simulink model "Ctrl_For_HRV"  (R2024b)
settings: Solver=ode4  StartTime=0.0  StopTime=100  FixedStep=0.02  RelTol=1e-3
InitFcn:
  | Parameter;
undefined symbols (not defined in the file or in its folder): CCI_DUI_AngleRate_Controller, CCI_DUI_FlowAngle_Controller, fhan, h_alpha, h_beta, h_miu, h_p, h_q, h_r, PNG_2026_6_24, r_alpha, r_beta, r_miu, r_p, r_q, r_r, xishu, xishu_D_0, xishu_L_0, xishu_l_0, xishu_m_0, xishu_n_0, xishu_Y_0
libraries: simulink x12
settings Model: Creator=BinRen  LastModifiedBy=DuY
settings SolverCC: AlgebraicLoopSolver=TrustRegion
settings DataIOCC: ReturnWorkspaceOutputs=off  TimeSaveName=time
settings DebuggingCC: UnconnectedInputMsg=warning  UnconnectedOutputMsg=warning  UnconnectedLineMsg=warning
settings ModelReferenceCC: EnableRefExpFcnMdlSchedulingChecks=on
settings RTWCC: GPUComputeCapability=3.5  DLArmComputeVersion=19.05

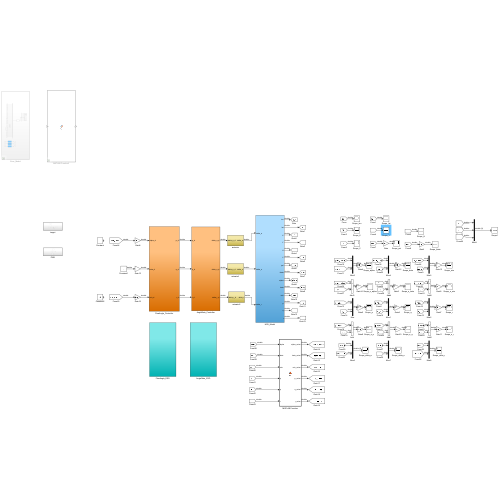
[thumbnail: Simulink's stored preview of the top-level diagram]
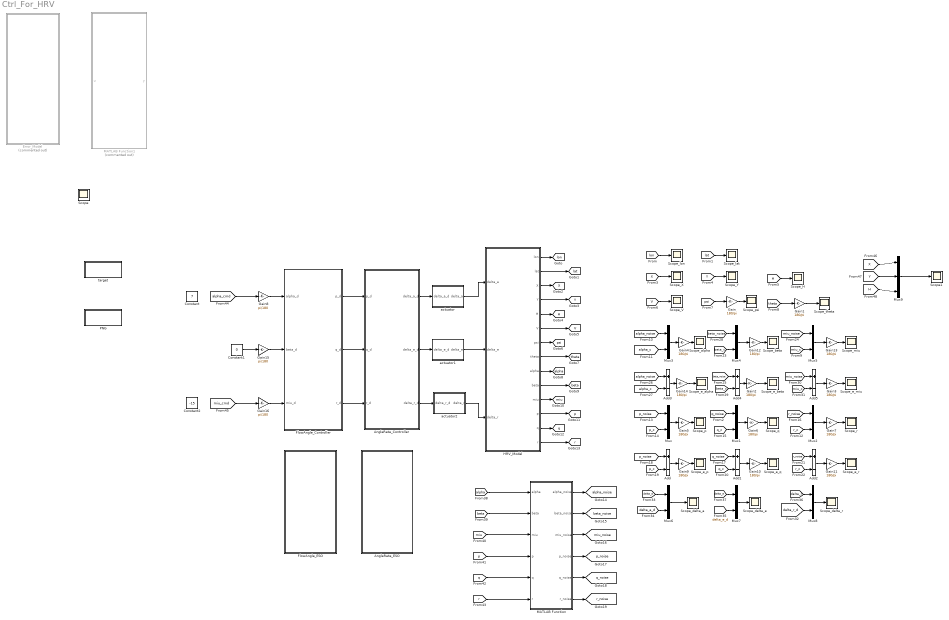
== system Ctrl_For_HRV ==
  Add{,1..5} (6 alike) : Sum  Inputs=+-
  AngleRate_Controller : Subsystem
  AngleRate_ESO : Subsystem
  Constant : Constant  Value=7  SampleTime=-1
  Constant1 : Constant  Value=0  SampleTime=-1
  Constant2 : Constant  Value=-15  SampleTime=-1
  Error_Model : Subsystem  Commented=on
  FlowAngle_Controller : Subsystem
  FlowAngle_ESO : Subsystem
  Gain{,1..7,9..14} (14 alike) : Gain  Gain=180/pi
  Gain15 : Gain  Gain=pi/180
  Gain16 : Gain  Gain=pi/180
  Gain8 : Gain  Gain=pi/180
  HRV_Model : Subsystem
  MATLAB Function : MATLAB Function  TreatAsAtomicUnit=on
  MATLAB Function1 : MATLAB Function  Commented=on  TreatAsAtomicUnit=on
  Mux{,1..8} (9 alike) : Mux  Inputs=2
  Mux9 : Mux  Inputs=3
  PNG : Subsystem
  Scope1 : Scope
  Scope_H : Scope
  Scope_V : Scope
  Scope_X : Scope
  Scope_Y : Scope
  Scope_alpha : Scope
  Scope_beta : Scope
  Scope_delta_a : Scope
  Scope_delta_e : Scope
  Scope_delta_r : Scope
  Scope_e_alpha : Scope
  Scope_e_beta : Scope
  Scope_e_miu : Scope
  Scope_e_p : Scope
  Scope_e_q : Scope
  Scope_e_r : Scope
  Scope_lat : Scope
  Scope_lon : Scope
  Scope_miu : Scope
  Scope_p : Scope
  Scope_psi : Scope
  Scope_q : Scope
  Scope_r : Scope
  Scope_theta : Scope
  actuator : Subsystem
  actuator1 : Subsystem
  actuator2 : Subsystem
  target : Subsystem
  Scope : Scope
  tag scope: H=global, V=global, X=global, Y=global, alpha=global, alpha_noise=global, beta=global, beta_noise=global, lat=global, lon=global, miu=global, miu_noise=global, p=global, p_noise=global, psi=global, q=global, q_noise=global, r=global, r_noise=global, theta=global
  wires:
  HRV_Model/1(lon) -> [lon]
  HRV_Model/2(lat) -> [lat]
  HRV_Model/4(Y) -> [Y]
  HRV_Model/3(X) -> [X]
  HRV_Model/7(psi) -> [psi]
  HRV_Model/8(theta) -> [theta]
  HRV_Model/6(V) -> [V]
  HRV_Model/5(H) -> [H]
  HRV_Model/13(q) -> [q]
  HRV_Model/14(r) -> [r]
  HRV_Model/11(miu) -> [miu]
  HRV_Model/12(p) -> [p]
  HRV_Model/10(beta) -> [beta]
  HRV_Model/9(alpha) -> [alpha]
  [lon] -> Scope_lon/1
  [lat] -> Scope_lat/1
  [H] -> Scope_H/1
  [Y] -> Scope_Y/1
  [X] -> Scope_X/1
  [V] -> Scope_V/1
  [psi] -> Gain/1
  Gain/1 -> Scope_psi/1
  Gain1/1 -> Scope_theta/1
  [theta] -> Gain1/1
  Gain5/1 -> Scope_p/1
  Gain6/1 -> Scope_q/1
  Gain7/1 -> Scope_r/1
  actuator/1(delta_a) -> HRV_Model/1(delta_a)
  actuator1/1(delta_e) -> HRV_Model/2(delta_e)
  actuator2/1(delta_r) -> HRV_Model/3(delta_r)
  AngleRate_Controller/2(delta_e_d) -> actuator1/1(delta_e_d)
  [p_noise] -> Mux/1
  Mux/1 -> Gain5/1
  [p_c] -> Mux/2
  [q_c] -> Mux1/2
  [q_noise] -> Mux1/1
  Mux1/1 -> Gain6/1
  Mux2/1 -> Gain7/1
  [r_noise] -> Mux2/1
  [r_c] -> Mux2/2
  Gain11/1 -> Scope_e_r/1
  Gain10/1 -> Scope_e_q/1
  Gain9/1 -> Scope_e_p/1
  [p_c] -> Add/2
  [p_noise] -> Add/1
  Add/1 -> Gain9/1
  Add1/1 -> Gain10/1
  [q_noise] -> Add1/1
  [q_c] -> Add1/2
  [r_c] -> Add2/2
  [r_noise] -> Add2/1
  Add2/1 -> Gain11/1
  Add5/1 -> Gain3/1
  [miu_noise] -> Add5/1
  [miu_c] -> Add5/2
  [beta_c] -> Add4/2
  [beta_noise] -> Add4/1
  Add4/1 -> Gain2/1
  Add3/1 -> Gain14/1
  [alpha_noise] -> Add3/1
  [alpha_c] -> Add3/2
  Gain14/1 -> Scope_e_alpha/1
  Gain2/1 -> Scope_e_beta/1
  Gain3/1 -> Scope_e_miu/1
  [miu_c] -> Mux5/2
  [miu_noise] -> Mux5/1
  Mux5/1 -> Gain13/1
  Mux4/1 -> Gain12/1
  [beta_noise] -> Mux4/1
  [beta_c] -> Mux4/2
  [alpha_c] -> Mux3/2
  Mux3/1 -> Gain4/1
  [alpha_noise] -> Mux3/1
  Gain13/1 -> Scope_miu/1
  Gain12/1 -> Scope_beta/1
  Gain4/1 -> Scope_alpha/1
  Gain8/1 -> FlowAngle_Controller/1(alpha_d)
  [delta_r_d] -> Mux8/2
  [delta_r] -> Mux8/1
  [delta_e] -> Mux7/1
  [delta_e_d] -> Mux7/2
  [delta_a_d] -> Mux6/2
  [delta_a] -> Mux6/1
  Mux8/1 -> Scope_delta_r/1
  Mux7/1 -> Scope_delta_e/1
  Mux6/1 -> Scope_delta_a/1
  FlowAngle_Controller/1(p_d) -> AngleRate_Controller/1(p_d)
  FlowAngle_Controller/2(q_d) -> AngleRate_Controller/2(q_d)
  FlowAngle_Controller/3(r_d) -> AngleRate_Controller/3(r_d)
  Constant1/1 -> Gain15/1
  Gain15/1 -> FlowAngle_Controller/2(beta_d)
  Gain16/1 -> FlowAngle_Controller/3(miu_d)
  AngleRate_Controller/3(delta_r_d) -> actuator2/1(delta_r_d)
  AngleRate_Controller/1(delta_a_d) -> actuator/1(delta_a_d)
  MATLAB Function/1(alpha_noise) -> [alpha_noise]
  [alpha] -> MATLAB Function/1(alpha)
  [beta] -> MATLAB Function/2(beta)
  [miu] -> MATLAB Function/3(miu)
  [p] -> MATLAB Function/4(p)
  [q] -> MATLAB Function/5(q)
  [r] -> MATLAB Function/6(r)
  MATLAB Function/2(beta_noise) -> [beta_noise]
  MATLAB Function/3(miu_noise) -> [miu_noise]
  MATLAB Function/4(p_noise) -> [p_noise]
  MATLAB Function/5(q_noise) -> [q_noise]
  MATLAB Function/6(r_noise) -> [r_noise]
  [miu_cmd] -> Gain16/1
  [alpha_cmd] -> Gain8/1
  [X] -> Mux9/1
  [Y] -> Mux9/2
  [H] -> Mux9/3
  Mux9/1 -> Scope1/1

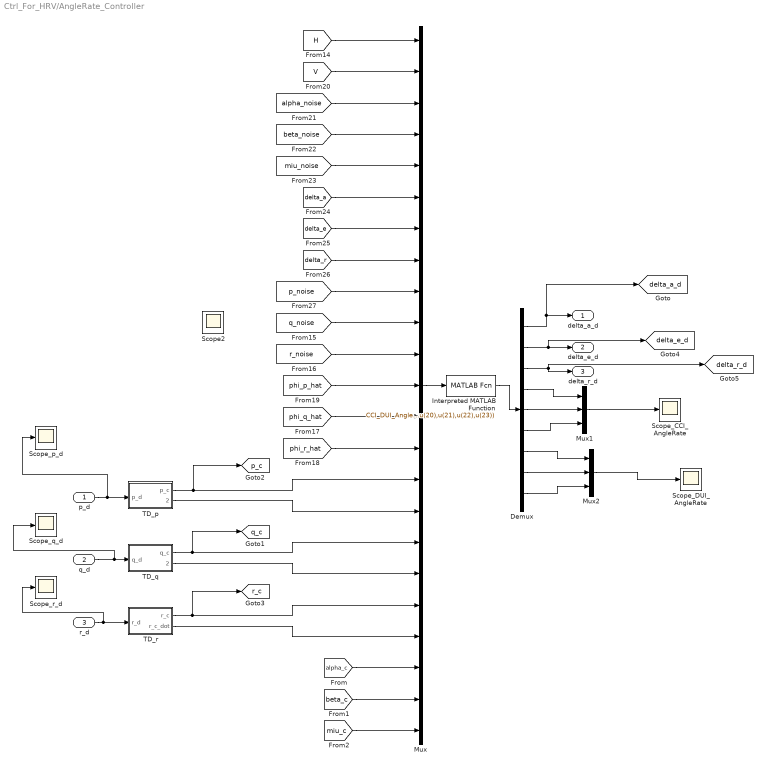
== system Ctrl_For_HRV/AngleRate_Controller ==
  p_d : Inport
  q_d : Inport  Port=2
  r_d : Inport  Port=3
  Demux : Demux  Outputs=9
  Interpreted MATLAB Function : MATLABFcn  MATLABFcn=CCI_DUI_AngleRate_Controller(u(1),u(2),u(3),u(4),u(5),u(6),u(7),u(8),u(9),u(10),u(11),u(12),u(13),u(14),u(15),u(16),u(17),u(18),u(19),u(20),u(21),u(22),u(23))  OutputDimensions=9
  Mux : Mux  Inputs=23
  Mux1 : Mux  Inputs=3
  Mux2 : Mux  Inputs=3
  Scope2 : Scope
  Scope_CCI_AngleRate : Scope
  Scope_DUI_AngleRate : Scope
  Scope_p_d : Scope
  Scope_q_d : Scope
  Scope_r_d : Scope
  TD_p : Subsystem
  TD_q : Subsystem
  TD_r : Subsystem
  delta_a_d : Outport
  delta_e_d : Outport  Port=2
  delta_r_d : Outport  Port=3
  tag scope: delta_a_d=global, delta_e_d=global, delta_r_d=global, p_c=global, q_c=global, r_c=global
  wires:
  [miu_noise] -> Mux/5
  [beta_noise] -> Mux/4
  TD_r/1(r_c) -> [r_c], Mux/19
  TD_p/2(p_c_dot) -> Mux/16
  TD_q/2(q_c_dot) -> Mux/18
  [q_noise] -> Mux/10
  TD_q/1(q_c) -> [q_c], Mux/17
  TD_r/2(r_c_dot) -> Mux/20
  [r_noise] -> Mux/11
  [H] -> Mux/1
  [p_noise] -> Mux/9
  [V] -> Mux/2
  [alpha_noise] -> Mux/3
  Mux/1 -> Interpreted MATLAB Function/1
  Interpreted MATLAB Function/1 -> Demux/1
  [delta_a] -> Mux/6
  [delta_r] -> Mux/8
  [delta_e] -> Mux/7
  TD_p/1(p_c) -> [p_c], Mux/15
  Demux/3 -> delta_r_d/1, [delta_r_d]
  r_d/1 -> Scope_r_d/1, TD_r/1(r_d)
  Demux/2 -> [delta_e_d], delta_e_d/1
  Demux/1 -> [delta_a_d], delta_a_d/1
  q_d/1 -> Scope_q_d/1, TD_q/1(q_d)
  p_d/1 -> Scope_p_d/1, TD_p/1(p_d)
  [phi_p_hat] -> Mux/12
  [phi_q_hat] -> Mux/13
  [phi_r_hat] -> Mux/14
  [alpha_c] -> Mux/21
  [beta_c] -> Mux/22
  [miu_c] -> Mux/23
  Demux/4 -> Mux1/1
  Demux/5 -> Mux1/2
  Demux/6 -> Mux1/3
  Mux1/1 -> Scope_CCI_AngleRate/1
  Demux/7 -> Mux2/1
  Demux/8 -> Mux2/2
  Demux/9 -> Mux2/3
  Mux2/1 -> Scope_DUI_AngleRate/1

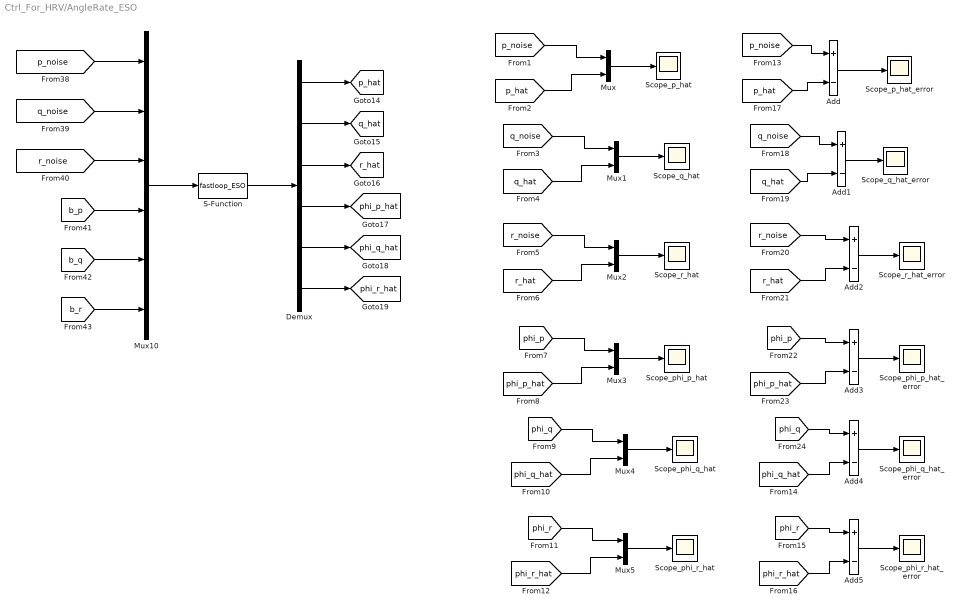
== system Ctrl_For_HRV/AngleRate_ESO ==
  Add{,1..5} (6 alike) : Sum  Inputs=+-
  Demux : Demux  Outputs=6
  Mux{,1..5} (6 alike) : Mux  Inputs=2
  Mux10 : Mux  Inputs=6
  S-Function : S-Function  FunctionName=fastloop_ESO  SFunctionDeploymentMode=off  EnableBusSupport=off
  Scope_p_hat : Scope
  Scope_p_hat_error : Scope
  Scope_phi_p_hat : Scope
  Scope_phi_p_hat_error : Scope
  Scope_phi_q_hat : Scope
  Scope_phi_q_hat_error : Scope
  Scope_phi_r_hat : Scope
  Scope_phi_r_hat_error : Scope
  Scope_q_hat : Scope
  Scope_q_hat_error : Scope
  Scope_r_hat : Scope
  Scope_r_hat_error : Scope
  tag scope: p_hat=global, phi_p_hat=global, phi_q_hat=global, phi_r_hat=global, q_hat=global, r_hat=global
  wires:
  [b_q] -> Mux10/5
  [r_noise] -> Mux10/3
  [q_noise] -> Mux10/2
  Demux/2 -> [q_hat]
  [b_p] -> Mux10/4
  S-Function/1 -> Demux/1
  Demux/5 -> [phi_q_hat]
  Demux/1 -> [p_hat]
  Demux/3 -> [r_hat]
  Demux/4 -> [phi_p_hat]
  Mux10/1 -> S-Function/1
  Demux/6 -> [phi_r_hat]
  [p_noise] -> Mux10/1
  [b_r] -> Mux10/6
  Mux/1 -> Scope_p_hat/1
  [p_noise] -> Mux/1
  [p_hat] -> Mux/2
  [q_noise] -> Mux1/1
  [q_hat] -> Mux1/2
  Mux1/1 -> Scope_q_hat/1
  [r_noise] -> Mux2/1
  [r_hat] -> Mux2/2
  Mux2/1 -> Scope_r_hat/1
  Mux5/1 -> Scope_phi_r_hat/1
  [phi_r_hat] -> Mux5/2
  [phi_r] -> Mux5/1
  Mux4/1 -> Scope_phi_q_hat/1
  [phi_q_hat] -> Mux4/2
  [phi_q] -> Mux4/1
  [phi_p_hat] -> Mux3/2
  [phi_p] -> Mux3/1
  Mux3/1 -> Scope_phi_p_hat/1
  [p_noise] -> Add/1
  [p_hat] -> Add/2
  Add/1 -> Scope_p_hat_error/1
  [q_noise] -> Add1/1
  [q_hat] -> Add1/2
  Add1/1 -> Scope_q_hat_error/1
  [r_noise] -> Add2/1
  [r_hat] -> Add2/2
  Add2/1 -> Scope_r_hat_error/1
  [phi_p] -> Add3/1
  [phi_p_hat] -> Add3/2
  Add3/1 -> Scope_phi_p_hat_error/1
  [phi_q] -> Add4/1
  [phi_q_hat] -> Add4/2
  Add4/1 -> Scope_phi_q_hat_error/1
  [phi_r] -> Add5/1
  [phi_r_hat] -> Add5/2
  Add5/1 -> Scope_phi_r_hat_error/1

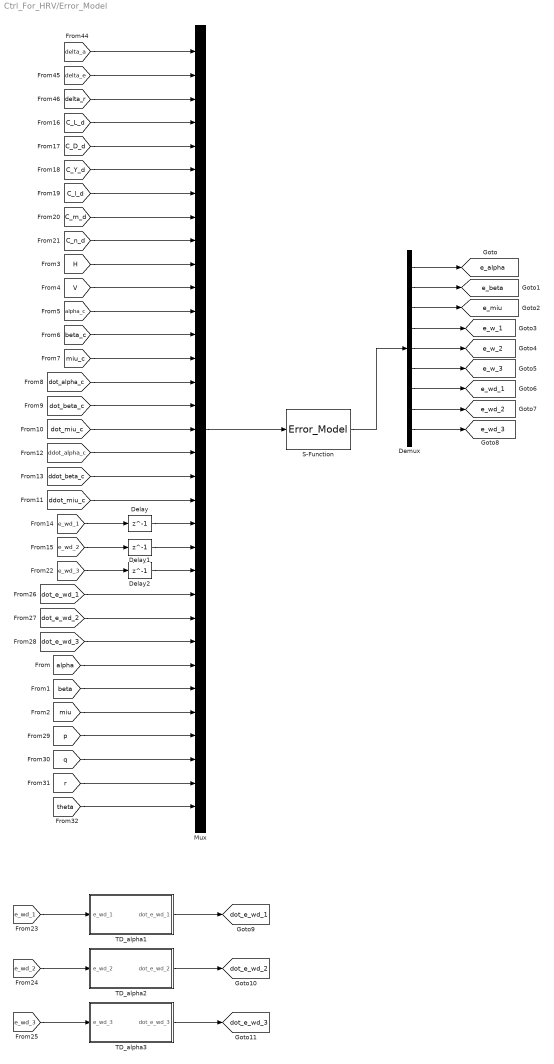
== system Ctrl_For_HRV/Error_Model ==
  Delay : Delay  DelayLength=1
  Delay1 : Delay  DelayLength=1
  Delay2 : Delay  DelayLength=1
  Demux : Demux  Outputs=9
  Mux : Mux  Inputs=33
  S-Function : S-Function  FunctionName=Error_Model  SFunctionDeploymentMode=off  EnableBusSupport=off
  TD_alpha1 : Subsystem
  TD_alpha2 : Subsystem
  TD_alpha3 : Subsystem
  tag scope: dot_e_wd_1=global, dot_e_wd_2=global, dot_e_wd_3=global, e_alpha=global, e_beta=global, e_miu=global, e_w_1=global, e_w_2=global, e_w_3=global, e_wd_1=global, e_wd_2=global, e_wd_3=global
  wires:
  Mux/1 -> S-Function/1
  [C_l_d] -> Mux/7
  [C_D_d] -> Mux/5
  [C_L_d] -> Mux/4
  [C_Y_d] -> Mux/6
  [C_n_d] -> Mux/9
  [C_m_d] -> Mux/8
  [H] -> Mux/10
  [V] -> Mux/11
  [alpha_c] -> Mux/12
  [beta_c] -> Mux/13
  [miu_c] -> Mux/14
  [dot_miu_c] -> Mux/17
  [dot_beta_c] -> Mux/16
  [dot_alpha_c] -> Mux/15
  [ddot_alpha_c] -> Mux/18
  [ddot_beta_c] -> Mux/19
  [ddot_miu_c] -> Mux/20
  S-Function/1 -> Demux/1
  Demux/1 -> [e_alpha]
  Demux/2 -> [e_beta]
  Demux/3 -> [e_miu]
  Demux/4 -> [e_w_1]
  Demux/5 -> [e_w_2]
  Demux/6 -> [e_w_3]
  Demux/9 -> [e_wd_3]
  Demux/8 -> [e_wd_2]
  Demux/7 -> [e_wd_1]
  [e_wd_1] -> Delay/1
  Delay/1 -> Mux/21
  Delay1/1 -> Mux/22
  [e_wd_2] -> Delay1/1
  [e_wd_3] -> Delay2/1
  Delay2/1 -> Mux/23
  [e_wd_1] -> TD_alpha1/1(e_wd_1)
  TD_alpha1/1(dot_e_wd_1) -> [dot_e_wd_1]
  TD_alpha2/1(dot_e_wd_2) -> [dot_e_wd_2]
  [e_wd_2] -> TD_alpha2/1(e_wd_2)
  [e_wd_3] -> TD_alpha3/1(e_wd_3)
  TD_alpha3/1(dot_e_wd_3) -> [dot_e_wd_3]
  [dot_e_wd_1] -> Mux/24
  [dot_e_wd_2] -> Mux/25
  [dot_e_wd_3] -> Mux/26
  [delta_a] -> Mux/1
  [delta_e] -> Mux/2
  [delta_r] -> Mux/3
  [alpha] -> Mux/27
  [beta] -> Mux/28
  [miu] -> Mux/29
  [p] -> Mux/30
  [q] -> Mux/31
  [r] -> Mux/32
  [theta] -> Mux/33

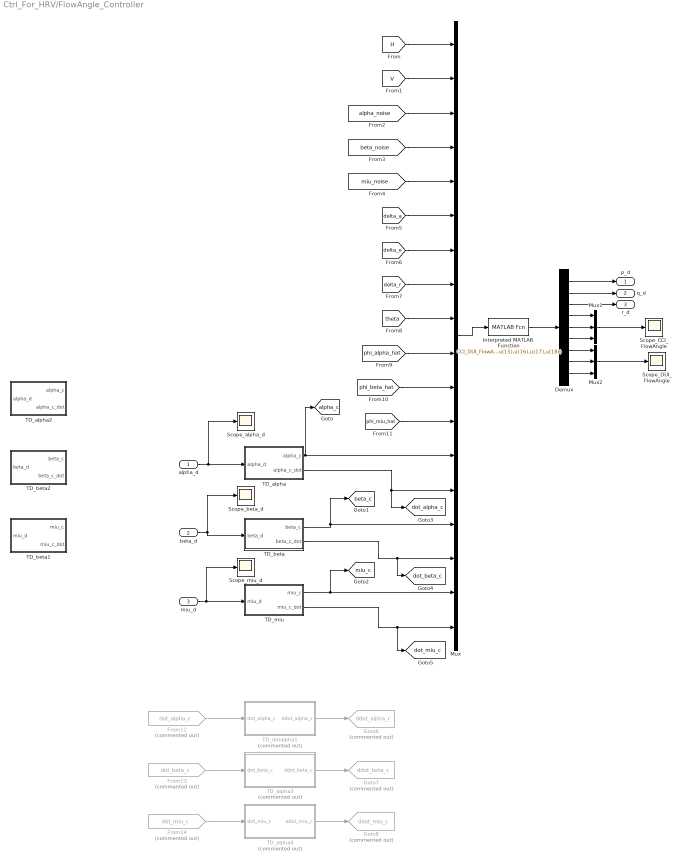
== system Ctrl_For_HRV/FlowAngle_Controller ==
  alpha_d : Inport
  beta_d : Inport  Port=2
  miu_d : Inport  Port=3
  Demux : Demux  Outputs=9
  From12 : From  Commented=on  GotoTag=dot_alpha_c  TagVisibility=global
  From13 : From  Commented=on  GotoTag=dot_beta_c  TagVisibility=global
  From14 : From  Commented=on  GotoTag=dot_miu_c  TagVisibility=global
  Goto6 : Goto  Commented=on  GotoTag=ddot_alpha_c  TagVisibility=global
  Goto7 : Goto  Commented=on  GotoTag=ddot_beta_c  TagVisibility=global
  Goto8 : Goto  Commented=on  GotoTag=ddot_miu_c  TagVisibility=global
  Interpreted MATLAB Function : MATLABFcn  MATLABFcn=CCI_DUI_FlowAngle_Controller(u(1),u(2),u(3),u(4),u(5),u(6),u(7),u(8),u(9),u(10),u(11),u(12),u(13),u(14),u(15),u(16),u(17),u(18))  OutputDimensions=9
  Mux : Mux  Inputs=18
  Mux1 : Mux  Inputs=3
  Mux2 : Mux  Inputs=3
  Scope_CCI_FlowAngle : Scope
  Scope_DUI_FlowAngle : Scope
  Scope_alpha_d : Scope
  Scope_beta_d : Scope
  Scope_miu_d : Scope
  TD_alpha : Subsystem
  TD_alpha2 : Subsystem
  TD_alpha3 : Subsystem  Commented=on
  TD_alpha4 : Subsystem  Commented=on
  TD_beta : Subsystem
  TD_beta1 : Subsystem
  TD_beta2 : Subsystem
  TD_dotalpha1 : Subsystem  Commented=on
  TD_miu : Subsystem
  p_d : Outport
  q_d : Outport  Port=2
  r_d : Outport  Port=3
  tag scope: alpha_c=global, beta_c=global, dot_alpha_c=global, dot_beta_c=global, dot_miu_c=global, miu_c=global
  wires:
  [H] -> Mux/1
  [V] -> Mux/2
  [alpha_noise] -> Mux/3
  [beta_noise] -> Mux/4
  [miu_noise] -> Mux/5
  [delta_r] -> Mux/8
  [delta_e] -> Mux/7
  [delta_a] -> Mux/6
  [theta] -> Mux/9
  Mux/1 -> Interpreted MATLAB Function/1
  Interpreted MATLAB Function/1 -> Demux/1
  Demux/1 -> p_d/1
  Demux/2 -> q_d/1
  Demux/3 -> r_d/1
  alpha_d/1 -> Scope_alpha_d/1, TD_alpha/1(alpha_d)
  TD_alpha/2(alpha_c_dot) -> Mux/14, [dot_alpha_c]
  beta_d/1 -> Scope_beta_d/1, TD_beta/1(beta_d)
  TD_beta/1(beta_c) -> [beta_c], Mux/15
  TD_beta/2(beta_c_dot) -> [dot_beta_c], Mux/16
  miu_d/1 -> Scope_miu_d/1, TD_miu/1(miu_d)
  TD_miu/1(miu_c) -> [miu_c], Mux/17
  TD_miu/2(miu_c_dot) -> [dot_miu_c], Mux/18
  [phi_alpha_hat] -> Mux/10
  [phi_beta_hat] -> Mux/11
  [phi_miu_hat] -> Mux/12
  From12/1 -> TD_dotalpha1/1(dot_alpha_c)
  TD_dotalpha1/1(ddot_alpha_c) -> Goto6/1
  From13/1 -> TD_alpha3/1(dot_beta_c)
  TD_alpha3/1(ddot_beta_c) -> Goto7/1
  From14/1 -> TD_alpha4/1(dot_miu_c)
  TD_alpha4/1(ddot_miu_c) -> Goto8/1
  TD_alpha/1(alpha_c) -> [alpha_c], Mux/13
  Demux/4 -> Mux1/1
  Demux/5 -> Mux1/2
  Demux/6 -> Mux1/3
  Mux1/1 -> Scope_CCI_FlowAngle/1
  Mux2/1 -> Scope_DUI_FlowAngle/1
  Demux/8 -> Mux2/2
  Demux/9 -> Mux2/3
  Demux/7 -> Mux2/1

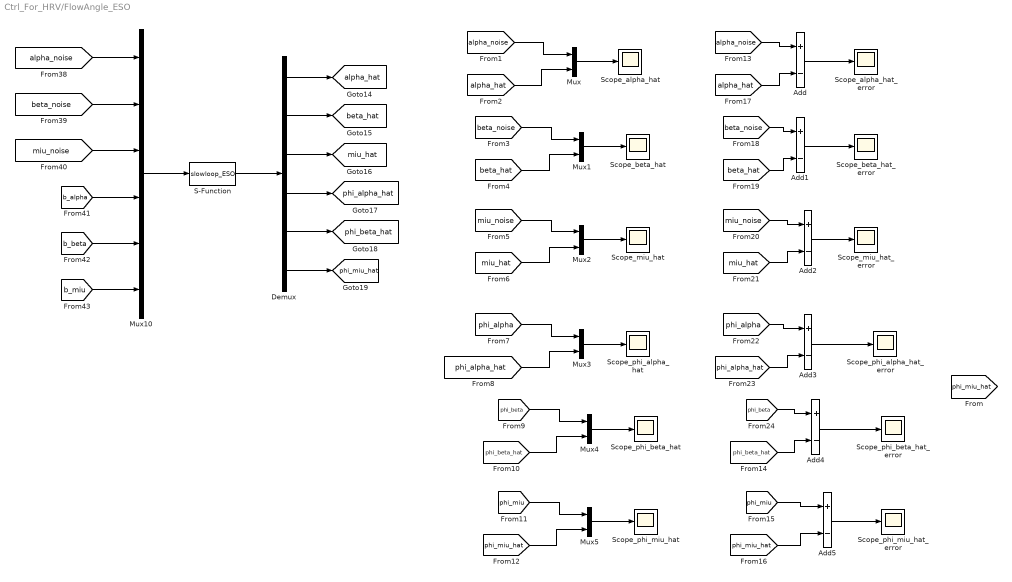
== system Ctrl_For_HRV/FlowAngle_ESO ==
  Add{,1..5} (6 alike) : Sum  Inputs=+-
  Demux : Demux  Outputs=6
  Mux{,1..5} (6 alike) : Mux  Inputs=2
  Mux10 : Mux  Inputs=6
  S-Function : S-Function  FunctionName=slowloop_ESO  SFunctionDeploymentMode=off  EnableBusSupport=off
  Scope_alpha_hat : Scope
  Scope_alpha_hat_error : Scope
  Scope_beta_hat : Scope
  Scope_beta_hat_error : Scope
  Scope_miu_hat : Scope
  Scope_miu_hat_error : Scope
  Scope_phi_alpha_hat : Scope
  Scope_phi_alpha_hat_error : Scope
  Scope_phi_beta_hat : Scope
  Scope_phi_beta_hat_error : Scope
  Scope_phi_miu_hat : Scope
  Scope_phi_miu_hat_error : Scope
  tag scope: alpha_hat=global, beta_hat=global, miu_hat=global, phi_alpha_hat=global, phi_beta_hat=global, phi_miu_hat=global
  wires:
  [b_beta] -> Mux10/5
  [miu_noise] -> Mux10/3
  [beta_noise] -> Mux10/2
  Demux/2 -> [beta_hat]
  [b_alpha] -> Mux10/4
  S-Function/1 -> Demux/1
  Demux/5 -> [phi_beta_hat]
  Demux/1 -> [alpha_hat]
  Demux/3 -> [miu_hat]
  Demux/4 -> [phi_alpha_hat]
  Mux10/1 -> S-Function/1
  Demux/6 -> [phi_miu_hat]
  [alpha_noise] -> Mux10/1
  [b_miu] -> Mux10/6
  Mux/1 -> Scope_alpha_hat/1
  [alpha_noise] -> Mux/1
  [alpha_hat] -> Mux/2
  [beta_noise] -> Mux1/1
  [beta_hat] -> Mux1/2
  Mux1/1 -> Scope_beta_hat/1
  [miu_noise] -> Mux2/1
  [miu_hat] -> Mux2/2
  Mux2/1 -> Scope_miu_hat/1
  Mux5/1 -> Scope_phi_miu_hat/1
  [phi_miu_hat] -> Mux5/2
  [phi_miu] -> Mux5/1
  Mux4/1 -> Scope_phi_beta_hat/1
  [phi_beta_hat] -> Mux4/2
  [phi_beta] -> Mux4/1
  [phi_alpha_hat] -> Mux3/2
  [phi_alpha] -> Mux3/1
  Mux3/1 -> Scope_phi_alpha_hat/1
  [alpha_noise] -> Add/1
  [alpha_hat] -> Add/2
  Add/1 -> Scope_alpha_hat_error/1
  [beta_noise] -> Add1/1
  [beta_hat] -> Add1/2
  Add1/1 -> Scope_beta_hat_error/1
  [miu_noise] -> Add2/1
  [miu_hat] -> Add2/2
  Add2/1 -> Scope_miu_hat_error/1
  [phi_alpha] -> Add3/1
  [phi_alpha_hat] -> Add3/2
  Add3/1 -> Scope_phi_alpha_hat_error/1
  [phi_beta] -> Add4/1
  [phi_beta_hat] -> Add4/2
  Add4/1 -> Scope_phi_beta_hat_error/1
  Add5/1 -> Scope_phi_miu_hat_error/1
  [phi_miu] -> Add5/1
  [phi_miu_hat] -> Add5/2

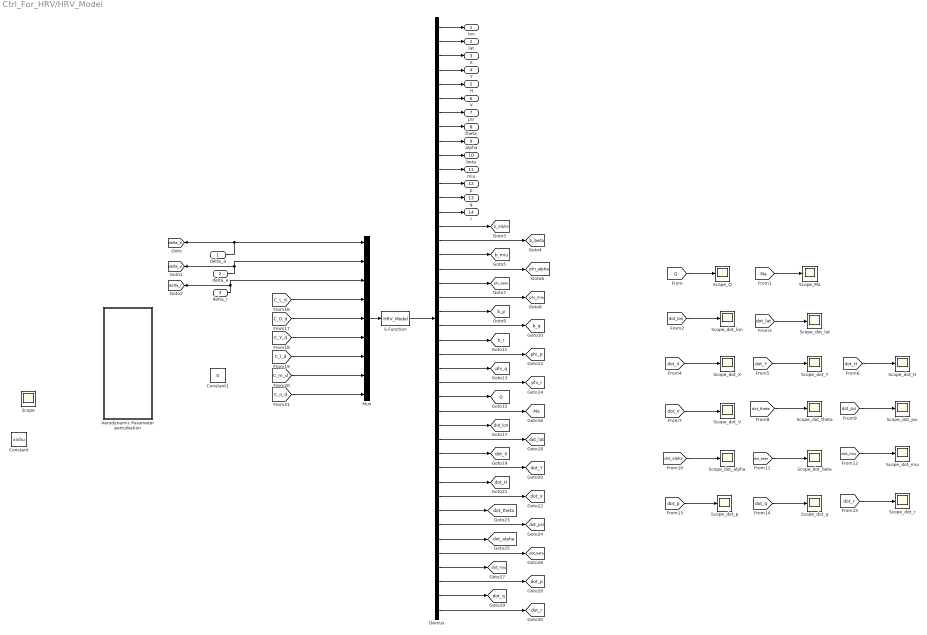
== system Ctrl_For_HRV/HRV_Model ==
  delta_a : Inport
  delta_e : Inport  Port=2
  delta_r : Inport  Port=3
  Aerodynamic Parameter perturbation : Subsystem
  Constant : Constant  Value=xishu  SampleTime=-1
  Constant1 : Constant  Value=0
  Demux : Demux  Outputs=14 + 12 + 2 + 14
  Mux : Mux  Inputs=9
  S-Function : S-Function  FunctionName=HRV_Model  SFunctionDeploymentMode=off  EnableBusSupport=off
  Scope : Scope
  Scope_Ma : Scope
  Scope_Q : Scope
  Scope_dot_H : Scope
  Scope_dot_V : Scope
  Scope_dot_X : Scope
  Scope_dot_Y : Scope
  Scope_dot_alpha : Scope
  Scope_dot_beta : Scope
  Scope_dot_lat : Scope
  Scope_dot_lon : Scope
  Scope_dot_miu : Scope
  Scope_dot_p : Scope
  Scope_dot_psi : Scope
  Scope_dot_q : Scope
  Scope_dot_r : Scope
  Scope_dot_theta : Scope
  lon : Outport
  lat : Outport  Port=2
  X : Outport  Port=3
  Y : Outport  Port=4
  H : Outport  Port=5
  V : Outport  Port=6
  psi : Outport  Port=7
  theta : Outport  Port=8
  alpha : Outport  Port=9
  beta : Outport  Port=10
  miu : Outport  Port=11
  p : Outport  Port=12
  q : Outport  Port=13
  r : Outport  Port=14
  tag scope: Ma=global, Q=global, b_alpha=global, b_beta=global, b_miu=global, b_p=global, b_q=global, b_r=global, delta_a=global, delta_e=global, delta_r=global, dot_H=global, dot_V=global, dot_X=global, dot_Y=global, dot_alpha=global, dot_beta=global, dot_lat=global, dot_lon=global, dot_miu=global, dot_p=global, dot_psi=global, dot_q=global, dot_r=global, dot_theta=global, phi_alpha=global, phi_beta=global, phi_miu=global, phi_p=global, phi_q=global, phi_r=global
  wires:
  Demux/8 -> theta/1
  Mux/1 -> S-Function/1
  S-Function/1 -> Demux/1
  Demux/1 -> lon/1
  Demux/2 -> lat/1
  Demux/3 -> X/1
  Demux/7 -> psi/1
  Demux/11 -> miu/1
  Demux/10 -> beta/1
  Demux/9 -> alpha/1
  Demux/12 -> p/1
  Demux/5 -> H/1
  delta_e/1 -> [delta_e], Mux/2
  Demux/6 -> V/1
  Demux/14 -> r/1
  delta_r/1 -> [delta_r], Mux/3
  Demux/13 -> q/1
  delta_a/1 -> [delta_a], Mux/1
  Demux/4 -> Y/1
  Demux/15 -> [b_alpha]
  Demux/16 -> [b_beta]
  Demux/18 -> [phi_alpha]
  Demux/17 -> [b_miu]
  Demux/21 -> [b_p]
  Demux/22 -> [b_q]
  Demux/20 -> [phi_miu]
  Demux/19 -> [phi_beta]
  Demux/23 -> [b_r]
  Demux/24 -> [phi_p]
  Demux/25 -> [phi_q]
  Demux/26 -> [phi_r]
  Demux/27 -> [Q]
  Demux/28 -> [Ma]
  Demux/30 -> [dot_lat]
  Demux/29 -> [dot_lon]
  Demux/31 -> [dot_X]
  Demux/32 -> [dot_Y]
  Demux/37 -> [dot_alpha]
  Demux/36 -> [dot_psi]
  Demux/34 -> [dot_V]
  Demux/35 -> [dot_theta]
  Demux/33 -> [dot_H]
  Demux/39 -> [dot_miu]
  Demux/38 -> [dot_beta]
  Demux/40 -> [dot_p]
  Demux/41 -> [dot_q]
  Demux/42 -> [dot_r]
  [Q] -> Scope_Q/1
  [Ma] -> Scope_Ma/1
  [dot_lon] -> Scope_dot_lon/1
  [dot_lat] -> Scope_dot_lat/1
  [dot_X] -> Scope_dot_X/1
  [dot_Y] -> Scope_dot_Y/1
  [dot_H] -> Scope_dot_H/1
  [dot_V] -> Scope_dot_V/1
  [dot_theta] -> Scope_dot_theta/1
  [dot_psi] -> Scope_dot_psi/1
  [dot_alpha] -> Scope_dot_alpha/1
  [dot_beta] -> Scope_dot_beta/1
  [dot_miu] -> Scope_dot_miu/1
  [dot_r] -> Scope_dot_r/1
  [dot_q] -> Scope_dot_q/1
  [dot_p] -> Scope_dot_p/1
  [C_L_d] -> Mux/4
  [C_D_d] -> Mux/5
  [C_Y_d] -> Mux/6
  [C_l_d] -> Mux/7
  [C_m_d] -> Mux/8
  [C_n_d] -> Mux/9

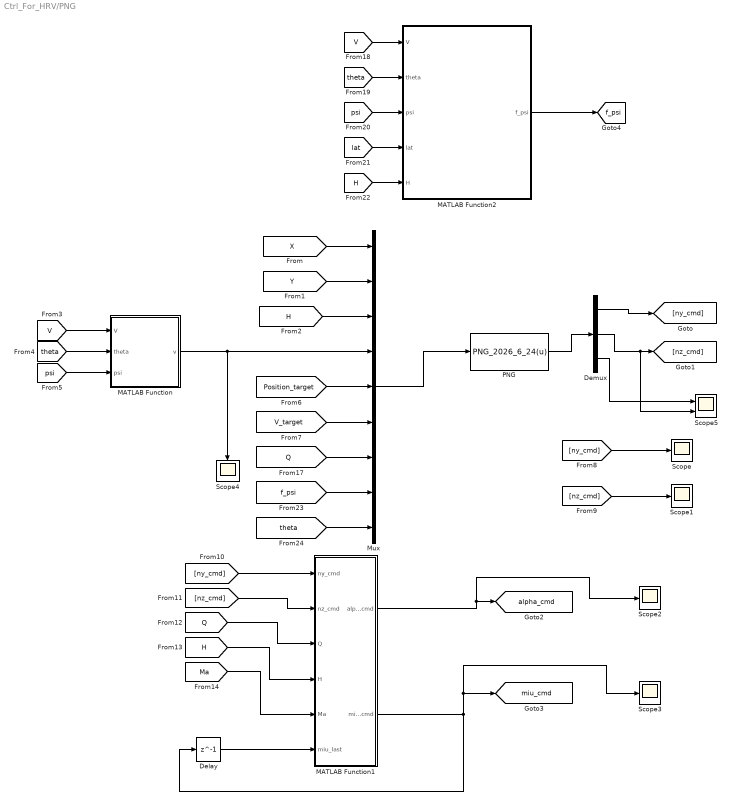
== system Ctrl_For_HRV/PNG ==
  Delay : Delay  DelayLength=1
  Demux : Demux  Outputs=3
  MATLAB Function : MATLAB Function  TreatAsAtomicUnit=on
  MATLAB Function1 : MATLAB Function  TreatAsAtomicUnit=on
  MATLAB Function2 : MATLAB Function  TreatAsAtomicUnit=on
  Mux : Mux  Inputs=7+2
  PNG : MATLABFcn  MATLABFcn=PNG_2026_6_24(u)  OutputDimensions=3
  Scope{,1..4} (5 alike) : Scope
  Scope5 : Scope  NumInputPorts=2
  tag scope: alpha_cmd=global, f_psi=global, miu_cmd=global
  wires:
  Mux/1 -> PNG/1
  [X] -> Mux/1
  [Y] -> Mux/2
  [H] -> Mux/3
  [V] -> MATLAB Function/1(V)
  [theta] -> MATLAB Function/2(theta)
  [psi] -> MATLAB Function/3(psi)
  MATLAB Function/1(v) -> Scope4/1, Mux/4
  [Position_target] -> Mux/5
  [V_target] -> Mux/6
  PNG/1 -> Demux/1
  Demux/1 -> [ny_cmd]
  Demux/2 -> Scope5/2, [nz_cmd]
  [ny_cmd] -> Scope/1
  [nz_cmd] -> Scope1/1
  [ny_cmd] -> MATLAB Function1/1(ny_cmd)
  [nz_cmd] -> MATLAB Function1/2(nz_cmd)
  [Q] -> MATLAB Function1/3(Q)
  [H] -> MATLAB Function1/4(H)
  [Ma] -> MATLAB Function1/5(Ma)
  MATLAB Function1/1(alpha_cmd) -> Scope2/1, [alpha_cmd]
  MATLAB Function1/2(miu_cmd) -> Delay/1, Scope3/1, [miu_cmd]
  [Q] -> Mux/7
  Demux/3 -> Scope5/1
  [V] -> MATLAB Function2/1(V)
  [theta] -> MATLAB Function2/2(theta)
  [psi] -> MATLAB Function2/3(psi)
  [lat] -> MATLAB Function2/4(lat)
  [H] -> MATLAB Function2/5(H)
  MATLAB Function2/1(f_psi) -> [f_psi]
  [f_psi] -> Mux/8
  [theta] -> Mux/9
  Delay/1 -> MATLAB Function1/6(miu_last)

== system Ctrl_For_HRV/actuator ==
  delta_a_d : Inport
  Gain : Gain  Gain=50
  Integrator : Integrator
  Saturation : Saturate  UpperLimit=90  LowerLimit=-90
  Saturation1 : Saturate  UpperLimit=30  LowerLimit=-30
  Sum : Sum  Inputs=|+-
  delta_a : Outport
  wires:
  Saturation/1 -> Integrator/1
  Sum/1 -> Gain/1
  Integrator/1 -> Saturation1/1, Sum/2
  delta_a_d/1 -> Sum/1
  Gain/1 -> Saturation/1
  Saturation1/1 -> delta_a/1

== system Ctrl_For_HRV/actuator1 ==
  delta_e_d : Inport
  Gain : Gain  Gain=50
  Integrator : Integrator
  Saturation : Saturate  UpperLimit=90  LowerLimit=-90
  Saturation1 : Saturate  UpperLimit=30  LowerLimit=-30
  Sum : Sum  Inputs=|+-
  delta_e : Outport
  wires:
  Saturation1/1 -> delta_e/1
  Gain/1 -> Saturation/1
  delta_e_d/1 -> Sum/1
  Integrator/1 -> Sum/2, Saturation1/1
  Sum/1 -> Gain/1
  Saturation/1 -> Integrator/1

== system Ctrl_For_HRV/actuator2 ==
  delta_r_d : Inport
  Gain : Gain  Gain=50
  Integrator : Integrator
  Saturation : Saturate  UpperLimit=90  LowerLimit=-90
  Saturation1 : Saturate  UpperLimit=30  LowerLimit=-30
  Sum : Sum  Inputs=|+-
  delta_r : Outport
  wires:
  Saturation/1 -> Integrator/1
  Sum/1 -> Gain/1
  Integrator/1 -> Saturation1/1, Sum/2
  delta_r_d/1 -> Sum/1
  Gain/1 -> Saturation/1
  Saturation1/1 -> delta_r/1

== system Ctrl_For_HRV/target ==
  Constant3 : Constant  Value=[0;0;0]
  Integrator : Integrator  InitialCondition=[500000;0;0]
  Scope1 : Scope
  tag scope: Position_target=global, V_target=global
  wires:
  Constant3/1 -> Integrator/1, [V_target]
  Integrator/1 -> [Position_target], Scope1/1

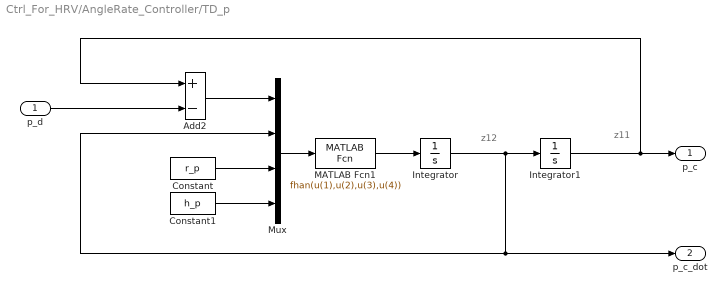
== system Ctrl_For_HRV/AngleRate_Controller/TD_p ==
  note: z11
  note: z12
  p_d : Inport
  Add2 : Sum  Inputs=+-
  Constant : Constant  Value=r_p
  Constant1 : Constant  Value=h_p
  Integrator : Integrator
  Integrator1 : Integrator
  MATLAB Fcn1 : MATLABFcn  MATLABFcn=fhan(u(1),u(2),u(3),u(4))
  Mux : Mux
  p_c : Outport  VectorParamsAs1DForOutWhenUnconnected=off
  p_c_dot : Outport  Port=2  VectorParamsAs1DForOutWhenUnconnected=off
  wires:
  Integrator/1 -> Integrator1/1, p_c_dot/1, Mux/2
  Integrator1/1 -> Add2/1, p_c/1
  MATLAB Fcn1/1 -> Integrator/1
  Mux/1 -> MATLAB Fcn1/1
  Constant/1 -> Mux/3
  Constant1/1 -> Mux/4
  Add2/1 -> Mux/1
  p_d/1 -> Add2/2

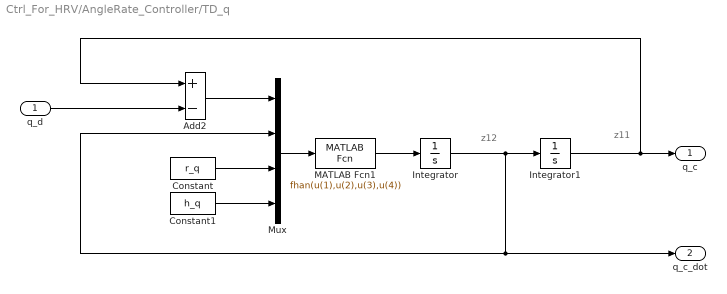
== system Ctrl_For_HRV/AngleRate_Controller/TD_q ==
  note: z11
  note: z12
  q_d : Inport
  Add2 : Sum  Inputs=+-
  Constant : Constant  Value=r_q
  Constant1 : Constant  Value=h_q
  Integrator : Integrator
  Integrator1 : Integrator
  MATLAB Fcn1 : MATLABFcn  MATLABFcn=fhan(u(1),u(2),u(3),u(4))
  Mux : Mux
  q_c : Outport  VectorParamsAs1DForOutWhenUnconnected=off
  q_c_dot : Outport  Port=2  VectorParamsAs1DForOutWhenUnconnected=off
  wires:
  Integrator/1 -> Integrator1/1, q_c_dot/1, Mux/2
  Integrator1/1 -> Add2/1, q_c/1
  MATLAB Fcn1/1 -> Integrator/1
  Mux/1 -> MATLAB Fcn1/1
  Constant/1 -> Mux/3
  Constant1/1 -> Mux/4
  Add2/1 -> Mux/1
  q_d/1 -> Add2/2

== system Ctrl_For_HRV/AngleRate_Controller/TD_r ==
  note: z11
  note: z12
  r_d : Inport
  Add2 : Sum  Inputs=+-
  Constant : Constant  Value=r_r
  Constant1 : Constant  Value=h_r
  Integrator : Integrator
  Integrator1 : Integrator
  MATLAB Fcn1 : MATLABFcn  MATLABFcn=fhan(u(1),u(2),u(3),u(4))
  Mux : Mux
  r_c : Outport  VectorParamsAs1DForOutWhenUnconnected=off
  r_c_dot : Outport  Port=2  VectorParamsAs1DForOutWhenUnconnected=off
  wires:
  Integrator/1 -> Integrator1/1, r_c_dot/1, Mux/2
  Integrator1/1 -> Add2/1, r_c/1
  MATLAB Fcn1/1 -> Integrator/1
  Mux/1 -> MATLAB Fcn1/1
  Constant/1 -> Mux/3
  Constant1/1 -> Mux/4
  Add2/1 -> Mux/1
  r_d/1 -> Add2/2

== system Ctrl_For_HRV/Error_Model/TD_alpha1 ==
  note: z11
  note: z12
  e_wd_1 : Inport
  Add2 : Sum  Inputs=+-
  Constant : Constant  Value=r_alpha
  Constant1 : Constant  Value=h_alpha
  Integrator : Integrator
  Integrator1 : Integrator
  MATLAB Fcn1 : MATLABFcn  MATLABFcn=fhan(u(1),u(2),u(3),u(4))
  Mux : Mux
  dot_e_wd_1 : Outport  VectorParamsAs1DForOutWhenUnconnected=off
  wires:
  Integrator/1 -> Integrator1/1, dot_e_wd_1/1, Mux/2
  Integrator1/1 -> Add2/1
  MATLAB Fcn1/1 -> Integrator/1
  Mux/1 -> MATLAB Fcn1/1
  Constant/1 -> Mux/3
  Constant1/1 -> Mux/4
  Add2/1 -> Mux/1
  e_wd_1/1 -> Add2/2

== system Ctrl_For_HRV/Error_Model/TD_alpha2 ==
  note: z12
  note: z11
  e_wd_2 : Inport
  Add2 : Sum  Inputs=+-
  Constant : Constant  Value=r_alpha
  Constant1 : Constant  Value=h_alpha
  Integrator : Integrator
  Integrator1 : Integrator
  MATLAB Fcn1 : MATLABFcn  MATLABFcn=fhan(u(1),u(2),u(3),u(4))
  Mux : Mux
  dot_e_wd_2 : Outport  VectorParamsAs1DForOutWhenUnconnected=off
  wires:
  e_wd_2/1 -> Add2/2
  Add2/1 -> Mux/1
  Constant1/1 -> Mux/4
  Constant/1 -> Mux/3
  Mux/1 -> MATLAB Fcn1/1
  MATLAB Fcn1/1 -> Integrator/1
  Integrator1/1 -> Add2/1
  Integrator/1 -> Mux/2, dot_e_wd_2/1, Integrator1/1

== system Ctrl_For_HRV/Error_Model/TD_alpha3 ==
  note: z11
  note: z12
  e_wd_3 : Inport
  Add2 : Sum  Inputs=+-
  Constant : Constant  Value=r_alpha
  Constant1 : Constant  Value=h_alpha
  Integrator : Integrator
  Integrator1 : Integrator
  MATLAB Fcn1 : MATLABFcn  MATLABFcn=fhan(u(1),u(2),u(3),u(4))
  Mux : Mux
  dot_e_wd_3 : Outport  VectorParamsAs1DForOutWhenUnconnected=off
  wires:
  Integrator/1 -> Integrator1/1, dot_e_wd_3/1, Mux/2
  Integrator1/1 -> Add2/1
  MATLAB Fcn1/1 -> Integrator/1
  Mux/1 -> MATLAB Fcn1/1
  Constant/1 -> Mux/3
  Constant1/1 -> Mux/4
  Add2/1 -> Mux/1
  e_wd_3/1 -> Add2/2

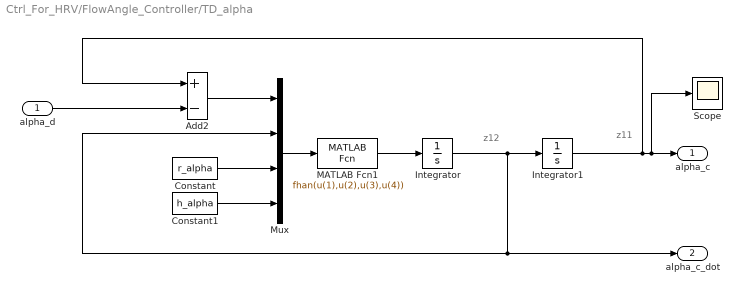
== system Ctrl_For_HRV/FlowAngle_Controller/TD_alpha ==
  note: z11
  note: z12
  alpha_d : Inport
  Add2 : Sum  Inputs=+-
  Constant : Constant  Value=r_alpha
  Constant1 : Constant  Value=h_alpha
  Integrator : Integrator
  Integrator1 : Integrator
  MATLAB Fcn1 : MATLABFcn  MATLABFcn=fhan(u(1),u(2),u(3),u(4))
  Mux : Mux
  Scope : Scope
  alpha_c : Outport  VectorParamsAs1DForOutWhenUnconnected=off
  alpha_c_dot : Outport  Port=2  VectorParamsAs1DForOutWhenUnconnected=off
  wires:
  Integrator/1 -> Integrator1/1, alpha_c_dot/1, Mux/2
  Integrator1/1 -> Add2/1, Scope/1, alpha_c/1
  MATLAB Fcn1/1 -> Integrator/1
  Mux/1 -> MATLAB Fcn1/1
  Constant/1 -> Mux/3
  Constant1/1 -> Mux/4
  Add2/1 -> Mux/1
  alpha_d/1 -> Add2/2

== system Ctrl_For_HRV/FlowAngle_Controller/TD_alpha2 ==
  alpha_d : Inport
  Gain17 : Gain  Gain=1.2
  Integrator : Integrator
  Sum : Sum  Inputs=|+-
  alpha_c : Outport
  alpha_c_dot : Outport  Port=2
  wires:
  Gain17/1 -> alpha_c_dot/1, Integrator/1
  Integrator/1 -> alpha_c/1, Sum/2
  Sum/1 -> Gain17/1
  alpha_d/1 -> Sum/1

== system Ctrl_For_HRV/FlowAngle_Controller/TD_alpha3 ==
  note: z11
  note: z12
  dot_beta_c : Inport
  Add2 : Sum  Inputs=+-
  Constant : Constant  Value=r_alpha
  Constant1 : Constant  Value=h_alpha
  Integrator : Integrator
  Integrator1 : Integrator
  MATLAB Fcn1 : MATLABFcn  MATLABFcn=fhan(u(1),u(2),u(3),u(4))
  Mux : Mux
  ddot_beta_c : Outport  VectorParamsAs1DForOutWhenUnconnected=off
  wires:
  Integrator/1 -> Integrator1/1, ddot_beta_c/1, Mux/2
  Integrator1/1 -> Add2/1
  MATLAB Fcn1/1 -> Integrator/1
  Mux/1 -> MATLAB Fcn1/1
  Constant/1 -> Mux/3
  Constant1/1 -> Mux/4
  Add2/1 -> Mux/1
  dot_beta_c/1 -> Add2/2

== system Ctrl_For_HRV/FlowAngle_Controller/TD_alpha4 ==
  note: z11
  note: z12
  dot_miu_c : Inport
  Add2 : Sum  Inputs=+-
  Constant : Constant  Value=r_alpha
  Constant1 : Constant  Value=h_alpha
  Integrator : Integrator
  Integrator1 : Integrator
  MATLAB Fcn1 : MATLABFcn  MATLABFcn=fhan(u(1),u(2),u(3),u(4))
  Mux : Mux
  ddot_miu_c : Outport  VectorParamsAs1DForOutWhenUnconnected=off
  wires:
  Integrator/1 -> Integrator1/1, ddot_miu_c/1, Mux/2
  Integrator1/1 -> Add2/1
  MATLAB Fcn1/1 -> Integrator/1
  Mux/1 -> MATLAB Fcn1/1
  Constant/1 -> Mux/3
  Constant1/1 -> Mux/4
  Add2/1 -> Mux/1
  dot_miu_c/1 -> Add2/2

== system Ctrl_For_HRV/FlowAngle_Controller/TD_beta ==
  note: z11
  note: z12
  beta_d : Inport
  Add2 : Sum  Inputs=+-
  Constant : Constant  Value=r_beta
  Constant1 : Constant  Value=h_beta
  Integrator : Integrator
  Integrator1 : Integrator
  MATLAB Fcn1 : MATLABFcn  MATLABFcn=fhan(u(1),u(2),u(3),u(4))
  Mux : Mux
  beta_c : Outport  VectorParamsAs1DForOutWhenUnconnected=off
  beta_c_dot : Outport  Port=2  VectorParamsAs1DForOutWhenUnconnected=off
  wires:
  Integrator/1 -> Integrator1/1, beta_c_dot/1, Mux/2
  Integrator1/1 -> Add2/1, beta_c/1
  MATLAB Fcn1/1 -> Integrator/1
  Mux/1 -> MATLAB Fcn1/1
  Constant/1 -> Mux/3
  Constant1/1 -> Mux/4
  Add2/1 -> Mux/1
  beta_d/1 -> Add2/2

== system Ctrl_For_HRV/FlowAngle_Controller/TD_beta1 ==
  miu_d : Inport
  Gain17 : Gain  Gain=0.8
  Integrator : Integrator
  Sum : Sum  Inputs=|+-
  miu_c : Outport
  miu_c_dot : Outport  Port=2
  wires:
  Gain17/1 -> miu_c_dot/1, Integrator/1
  Integrator/1 -> miu_c/1, Sum/2
  Sum/1 -> Gain17/1
  miu_d/1 -> Sum/1

== system Ctrl_For_HRV/FlowAngle_Controller/TD_beta2 ==
  beta_d : Inport
  Gain17 : Gain  Gain=1.2
  Integrator : Integrator
  Sum : Sum  Inputs=|+-
  beta_c : Outport
  beta_c_dot : Outport  Port=2
  wires:
  beta_d/1 -> Sum/1
  Sum/1 -> Gain17/1
  Integrator/1 -> Sum/2, beta_c/1
  Gain17/1 -> Integrator/1, beta_c_dot/1

== system Ctrl_For_HRV/FlowAngle_Controller/TD_dotalpha1 ==
  note: z11
  note: z12
  dot_alpha_c : Inport
  Add2 : Sum  Inputs=+-
  Constant : Constant  Value=r_alpha
  Constant1 : Constant  Value=h_alpha
  Integrator : Integrator
  Integrator1 : Integrator
  MATLAB Fcn1 : MATLABFcn  MATLABFcn=fhan(u(1),u(2),u(3),u(4))
  Mux : Mux
  ddot_alpha_c : Outport  VectorParamsAs1DForOutWhenUnconnected=off
  wires:
  Integrator/1 -> Integrator1/1, ddot_alpha_c/1, Mux/2
  Integrator1/1 -> Add2/1
  MATLAB Fcn1/1 -> Integrator/1
  Mux/1 -> MATLAB Fcn1/1
  Constant/1 -> Mux/3
  Constant1/1 -> Mux/4
  Add2/1 -> Mux/1
  dot_alpha_c/1 -> Add2/2

== system Ctrl_For_HRV/FlowAngle_Controller/TD_miu ==
  note: z11
  note: z12
  miu_d : Inport
  Add2 : Sum  Inputs=+-
  Constant : Constant  Value=r_miu
  Constant1 : Constant  Value=h_miu
  Integrator : Integrator
  Integrator1 : Integrator
  MATLAB Fcn1 : MATLABFcn  MATLABFcn=fhan(u(1),u(2),u(3),u(4))
  Mux : Mux
  miu_c : Outport  VectorParamsAs1DForOutWhenUnconnected=off
  miu_c_dot : Outport  Port=2  VectorParamsAs1DForOutWhenUnconnected=off
  wires:
  Integrator/1 -> Integrator1/1, miu_c_dot/1, Mux/2
  Integrator1/1 -> Add2/1, miu_c/1
  MATLAB Fcn1/1 -> Integrator/1
  Mux/1 -> MATLAB Fcn1/1
  Constant/1 -> Mux/3
  Constant1/1 -> Mux/4
  Add2/1 -> Mux/1
  miu_d/1 -> Add2/2

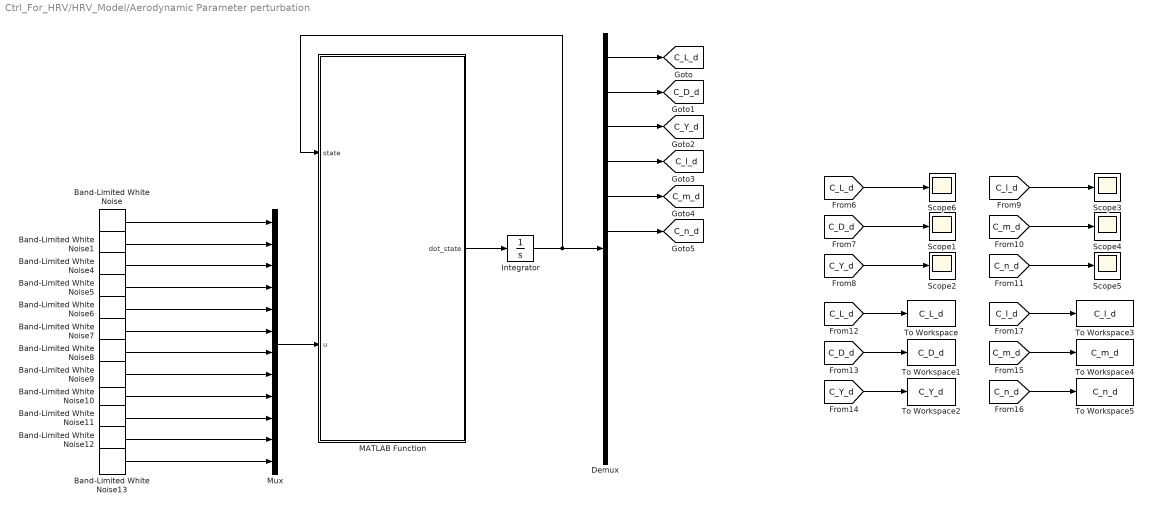
== system Ctrl_For_HRV/HRV_Model/Aerodynamic Parameter perturbation ==
  Band-Limited White Noise{,1,4..7} (6 alike) : simulink/Sources/Band-Limited White Noise  Cov=1e-6  Ts=2  seed=round(rand()*1e5)
  Band-Limited White Noise{8..13} (6 alike) : simulink/Sources/Band-Limited White Noise  Cov=1e-10  Ts=2  seed=round(rand()*1e5)
  Demux : Demux  Outputs=12
  Integrator : Integrator  InitialCondition=[xishu_L_0,xishu_D_0,xishu_Y_0,xishu_l_0,xishu_m_0,xishu_n_0,0,0,0,0,0,0]
  MATLAB Function : MATLAB Function  TreatAsAtomicUnit=on
  Mux : Mux  Inputs=12
  Scope{1..6} (6 alike) : Scope
  To Workspace : ToWorkspace  VariableName=C_L_d  SampleTime=-1
      settings: Save2DSignal=2-D array (concatenate along first dimension)
  To Workspace1 : ToWorkspace  VariableName=C_D_d  SampleTime=-1
      settings: Save2DSignal=2-D array (concatenate along first dimension)
  To Workspace2 : ToWorkspace  VariableName=C_Y_d  SampleTime=-1
      settings: Save2DSignal=2-D array (concatenate along first dimension)
  To Workspace3 : ToWorkspace  VariableName=C_l_d  SampleTime=-1
      settings: Save2DSignal=2-D array (concatenate along first dimension)
  To Workspace4 : ToWorkspace  VariableName=C_m_d  SampleTime=-1
      settings: Save2DSignal=2-D array (concatenate along first dimension)
  To Workspace5 : ToWorkspace  VariableName=C_n_d  SampleTime=-1
      settings: Save2DSignal=2-D array (concatenate along first dimension)
  tag scope: C_D_d=global, C_L_d=global, C_Y_d=global, C_l_d=global, C_m_d=global, C_n_d=global
  wires:
  Mux/1 -> MATLAB Function/2(u)
  Band-Limited White Noise/1 -> Mux/1
  Band-Limited White Noise1/1 -> Mux/2
  Band-Limited White Noise5/1 -> Mux/4
  Band-Limited White Noise4/1 -> Mux/3
  Band-Limited White Noise6/1 -> Mux/5
  Band-Limited White Noise7/1 -> Mux/6
  Band-Limited White Noise8/1 -> Mux/7
  Band-Limited White Noise9/1 -> Mux/8
  Band-Limited White Noise10/1 -> Mux/9
  Band-Limited White Noise11/1 -> Mux/10
  Band-Limited White Noise12/1 -> Mux/11
  Band-Limited White Noise13/1 -> Mux/12
  MATLAB Function/1(dot_state) -> Integrator/1
  Integrator/1 -> Demux/1, MATLAB Function/1(state)
  Demux/1 -> [C_L_d]
  Demux/2 -> [C_D_d]
  Demux/3 -> [C_Y_d]
  Demux/4 -> [C_l_d]
  Demux/5 -> [C_m_d]
  Demux/6 -> [C_n_d]
  [C_Y_d] -> Scope2/1
  [C_m_d] -> Scope4/1
  [C_n_d] -> Scope5/1
  [C_l_d] -> Scope3/1
  [C_L_d] -> Scope6/1
  [C_D_d] -> Scope1/1
  [C_D_d] -> To Workspace1/1
  [C_L_d] -> To Workspace/1
  [C_Y_d] -> To Workspace2/1
  [C_l_d] -> To Workspace3/1
  [C_m_d] -> To Workspace4/1
  [C_n_d] -> To Workspace5/1

== matlab function Ctrl_For_HRV/MATLAB Function ==
  settings: updateMethod=DISCRETE
  data: alpha input; alpha_noise output; beta input; miu input; p input; q input; r input; beta_noise output; miu_noise output; p_noise output; q_noise output; r_noise output
function [alpha_noise,beta_noise,miu_noise,p_noise,q_noise,r_noise]= fcn(alpha,beta,miu,p,q,r)

% alpha_noise = awgn(alpha,100);
% beta_noise = awgn(beta,100);
% miu_noise = awgn(miu,100);
% p_noise = awgn(p,100);
% q_noise = awgn(q,100);
% r_noise = awgn(r,100);

alpha_noise = alpha;
beta_noise = beta;
miu_noise = miu;
p_noise = p;
q_noise = q;
r_noise = r;

== matlab function Ctrl_For_HRV/HRV_Model/Aerodynamic Parameter perturbation/MATLAB Function ==
  data: state input; dot_state output; u input
function dot_state  = Shedong_Model(state,u)
    C_L_d = state(1);C_D_d = state(2);C_Y_d = state(3);C_l_d = state(4);C_m_d = state(5);C_n_d = state(6);
    xi_L = state(7);xi_D = state(8);xi_Y = state(9);xi_l = state(10);xi_m = state(11);xi_n = state(12);
    omega_C_L_d = u(1);omega_C_D_d = u(2);omega_C_Y_d = u(3);omega_C_l_d = u(4);omega_C_m_d = u(5);omega_C_n_d = u(6);
    omega_xi_L_d = u(7);omega_xi_D_d = u(8);omega_xi_Y_d = u(9);omega_xi_l_d = u(10);omega_xi_m_d = u(11);omega_xi_n_d = u(12);

    dot_C_L_d = -xi_L*C_L_d+omega_C_L_d;    
    dot_C_D_d = -xi_D*C_D_d+omega_C_D_d;
    dot_C_Y_d = -xi_Y*C_Y_d+omega_C_Y_d;
    dot_C_l_d = -xi_l*C_l_d+omega_C_l_d;
    dot_C_m_d = -xi_m*C_m_d+omega_C_m_d;
    dot_C_n_d = -xi_n*C_n_d+omega_C_n_d;
    dot_xi_L = omega_xi_L_d;
    dot_xi_D = omega_xi_D_d;
    dot_xi_Y = omega_xi_Y_d;
    dot_xi_l = omega_xi_l_d;
    dot_xi_m = omega_xi_m_d;
    dot_xi_n = omega_xi_n_d;
            
    dot_state = [dot_C_L_d,dot_C_D_d,dot_C_Y_d,dot_C_l_d,dot_C_m_d,dot_C_n_d,dot_xi_L,dot_xi_D,dot_xi_Y,dot_xi_l,dot_xi_m,dot_xi_n];
end

== matlab function Ctrl_For_HRV/MATLAB Function1 ==
  data: u input; y output
function y = fcn(u)

omega_c = [alpha_c;beta_c;miu_c];
dot_omega_c = [dot_alpha_c;dot_beta_c;dot_miu_c];
ddot_omega_c = [ddot_alpha_c;ddot_beta_c;ddot_miu_c];
e_wd = [e_wd_1;e_wd_2;e_wd_3];
dot_e_wd = [dot_e_wd_1;dot_e_wd_2;dot_e_wd_3];

[Ma,Q] = M_Q(H,V);
%计算气动系数
[C_L_alpha,C_L_delta_a,C_L_delta_e] = Coefficient_Lift(alpha,Ma,delta_a,delta_e,delta_r);
[C_D_alpha,C_D_delta_a,C_D_delta_e,C_D_delta_r] = Coefficient_Drag(alpha,Ma,delta_a,delta_e,delta_r);
[C_Y_beta,C_Y_delta_a,C_Y_delta_e,C_Y_delta_r] = Coefficient_Side(alpha,Ma,delta_a,delta_e,delta_r);
% [C_L_alpha,C_L_delta_a,C_L_delta_e] = Coefficient_Lift(alpha,Ma,0,0,0);
% [C_D_alpha,C_D_delta_a,C_D_delta_e,C_D_delta_r] = Coefficient_Drag(alpha,Ma,0,0,0);
% [C_Y_beta,C_Y_delta_a,C_Y_delta_e,C_Y_delta_r] = Coefficient_Side(alpha,Ma,0,0,0);
[C_l_beta,C_l_delta_a,C_l_delta_e,C_l_delta_r,C_l_r,C_l_p] = Coefficient_RollingMoment(alpha,Ma,delta_a,delta_e,delta_r);
[C_m_alpha,C_m_delta_a,C_m_delta_e,C_m_delta_r,C_m_q] = Coefficient_PitchMoment(alpha,Ma,delta_a,delta_e,delta_r);
[C_n_beta,C_n_delta_a,C_n_delta_e,C_n_delta_r,C_n_p,C_n_r] = Coefficient_YawingMoment(alpha,Ma,delta_a,delta_e,delta_r);
C_L = C_L_alpha+C_L_delta_a+C_L_delta_e;
C_D = C_D_alpha+C_D_delta_a+C_D_delta_e+C_D_delta_r;
C_Y = C_Y_beta*beta+C_Y_delta_a+C_Y_delta_e+C_Y_delta_r;
C_l = C_l_beta*beta+C_l_delta_a*delta_a+C_l_delta_e*delta_e+C_l_delta_r*delta_r+C_l_r*(r*b/(2*V))+C_l_p*(p*b/(2*V));
C_m = C_m_alpha+C_m_delta_a*delta_a+C_m_delta_e*delta_e+C_m_delta_r*delta_r+C_m_q*(q*c/(2*V));
C_n = C_n_beta*beta+C_n_delta_a*delta_a+C_n_delta_e*delta_e+C_n_delta_r*delta_r+C_n_p*(p*b/(2*V))+C_n_r*(r*b/(2*V));

%摄动值
Delta_C_L = C_L_d*C_L; Delta_C_D = C_D_d*C_D; Delta_C_Y = C_Y_d*C_Y;
Delta_C_l = C_l_d*C_l; Delta_C_m = C_m_d*C_m; Delta_C_n = C_n_d*C_n;

%%重力加速度
R = earth_r+H; %R为地心距
g = (earth_r/R)^2*g0;

%%
% 模型调整
%先得到系数
Coefficient_C_L_alpha = 1.86e-2 + 1.01e-4 + 1.01e-4;
C_L_else = C_L - Coefficient_C_L_alpha * alpha;

Coefficient_C_Y_alpha = -1.12e-7 + 1.12e-7 + 4.86e-20;
C_Y_else = C_Y - Coefficient_C_Y_alpha * alpha;

Coefficient_C_l_beta_0 = -1.402e-1;
C_l_beta_else = C_l_beta - Coefficient_C_l_beta_0;

Coefficient_C_l_p_0 = -2.99e-1;
C_l_p_else = C_l_p - Coefficient_C_l_p_0;

Coefficient_C_l_r_0 = 3.82e-1;
C_l_r_else = C_l_r - Coefficient_C_l_r_0;

Coefficient_C_m_alpha_alpha = -2.260e-3 -6.59e-5 -6.59e-5;
C_m_alpha_else = C_m_alpha - Coefficient_C_m_alpha_alpha*alpha;

Coefficient_C_m_q_0 = -1.36;
C_m_q_else = C_m_q - Coefficient_C_m_q_0;

Coefficient_C_n_p_0 = 3.68e-1;
C_n_p_else = C_n_p - Coefficient_C_n_p_0;


%将模改写为面向控制的形式
d_alpha = 0.1*0.005*sin(0.2*pi*t); d_beta = 0.1*0.005*sin(0.2*pi*t); d_miu = 0.1*0.005*sin(0.2*pi*t);
d_p = 0.1*0.007*sin(pi*t); d_q = 0.1*0.01*sin(pi*t); d_r = 0;
%姿态角环
omega = [alpha;beta;miu];
w = [p;q;r];
u = [delta_a;delta_e;delta_r];

W_oo = [-Q*S*Coefficient_C_L_alpha,0,0;
        Q*S*Coefficient_C_Y_alpha,0,0;
        Q*S*(Coefficient_C_L_alpha*(tan(theta)*sin(miu)+tan(beta))+Coefficient_C_Y_alpha*tan(theta)*cos(beta)*cos(miu))];
F_else = [-Q*S*C_L_else,0,0;
        Q*S*C_Y_else,0,0;
        Q*S*(C_L_else*(tan(theta)*sin(miu)+tan(beta))+C_Y_else*tan(theta)*cos(beta)*cos(miu))];
f_o = [(m*g*cos(theta)*cos(miu))/(m*V*cos(beta));
       (m*g*cos(theta)*sin(miu))/(m*V);
       (-m*g*cos(theta)*tan(beta)*cos(miu))/(m*V)];
g_o = [-p*cos(alpha)*tan(beta) - r*sin(alpha)*tan(beta);
       p*sin(alpha);
       r*sin(alpha)*sec(beta)];
W_ow = [0,1,0;
        0,0,-cos(alpha);
        cos(alpha)*sec(beta)];
phi_s = [(-Q*S*Delta_C_L)/(m*V*cos(beta))+d_alpha;
         (Q*S*Delta_C_Y)/(m*V)+d_beta;
         (Q*S*Delta_C_L*(tan(theta)*sin(miu)+tan(beta))+Q*S*Delta_C_Y*tan(theta)*cos(beta)*cos(miu))/(m*V)+d_miu];
D_F = f_o + F_else + phi_s;
Dot_o = W_oo*omega + W_ow*w + g_o + D_F;

%角速度环
W_wo = [0,Q*S*b*Coefficient_C_l_beta_0/I_xx,0;
        Q*S*c_A*Coefficient_C_m_alpha_alpha/I_yy,0,0;
        0,0,0];
W_ww = [(Q*S*b/I_xx)*(Coefficient_C_l_p_0*b/(2*V)),0,(Q*S*b/I_xx)*(Coefficient_C_l_r_0*b/(2*V));
        0,(Q*S*c_A/I_yy)*Coefficient_C_m_q_0*c_A/(2*V),0;
        (Q*S*b/I_zz)*Coefficient_C_n_p_0*b/(2*V),0,0];
M_else = [(Q*S*b/I_xx)*(C_l_beta_else*beta+C_l_p_else*(p*b/(2*V))+C_l_r_else*(r*b/(2*V)));
          (Q*S*c_A/I_yy)*(C_m_alpha_else+C_m_q_else*(q*c_A/(2*V)));
          (Q*S*b/I_zz)*(C_n_beta*beta+C_n_p_else*(p*b/(2*V))+C_n_r*(r*b/(2*V)))];
f_w = [(I_yy-I_zz)*q*r/I_xx;
       (I_zz-I_xx)*p*r/I_yy;
       (I_xx-I_yy)*p*q/I_zz];
g_f = [Q*S*b*C_l_delta_a/I_xx   Q*S*b*C_l_delta_e/I_xx   Q*S*b*C_l_delta_r/I_xx;
       Q*S*c_A*C_m_delta_a/I_yy Q*S*c_A*C_m_delta_e/I_yy Q*S*c_A*C_m_delta_r/I_yy;
       Q*S*b*C_n_delta_a/I_zz   Q*S*b*C_n_delta_e/I_zz   Q*S*b*C_n_delta_r/I_zz];
phi_f = [Q*S*b*Delta_C_l/I_xx+d_p;
         Q*S*c_A*Delta_C_m/I_yy+d_q;
         Q*S*b*Delta_C_n/I_zz+d_r];
D_M = M_else + phi_f;

Dot_w = W_ww*w + W_wo*omega + g_f*u + f_w + D_M;
%%
%计算误差系统
%e_omega = omega - omega_c;
%e_w = W_ow*w + W_oo*omega_c - dot_omega_c - e_wd;

A_oo = W_oo;
A_ww = W_ow*W_ww*inv(W_ow);
A_wo = W_ow*W_wo;
B = W_ow*g_f;
h = (W_ow*W_wo - W_ow*W_ww*inv(W_ow)*W_oo)*omega_c + (W_oo+W_ow*W_ww*inv(W_ow))*dot_omega_c - ddot_omega_c;
r = W_ow*W_ww*inv(W_ow)*e_wd - dot_e_wd;
D_M_error = W_ow*D_M;

dot_e_omega = A_oo*e_omega + e_w + e_wd + g_o + D_F;
dot_e_w = A_ww*e_w + A_wo*e_omega + f_w + B*u + h + r + D_M_error;


dot_error_alpha = dot_e_omega(1); dot_error_beta = dot_e_omega(2); dot_error_miu = dot_e_omega(3);
dot_error_w_1 = dot_e_w(1); dot_error_w_2 = dot_e_w(2); dot_error_w_3 = dot_e_w(3);

x_dot=[dot_error_alpha;dot_error_beta;dot_error_miu;dot_error_w_1;dot_error_w_2;dot_error_w_3];
sys = x_dot;



y = u;

== matlab function Ctrl_For_HRV/PNG/MATLAB Function ==
  data: V input; v output; theta input; psi input
function v = fcn(V,theta,psi)
dot_X = V*cos(theta)*cos(psi);
dot_Y = V*cos(theta)*sin(psi);
dot_H = V*sin(theta);

v=[dot_X;dot_Y;dot_H];

== matlab function Ctrl_For_HRV/PNG/MATLAB Function1 ==
  data: ny_cmd input; alpha_cmd output; nz_cmd input; miu_cmd output; Q input; H input; Ma input; miu_last input
function [alpha_cmd, miu_cmd] = fcn(ny_cmd,nz_cmd,Q, H, Ma, miu_last)
%%%%%%%%%该函数的作用为将过载指令转化为攻角指令与倾侧角指令
%%
%参数设置
S = 334.73;
m = 63504;
earth_r = 6371000;
g0 = 9.8060;
R = earth_r+H; %R为地心距
g = (earth_r/R)^2*g0;
%% ===== 倾侧角 =====
nL=sqrt(ny_cmd^2+nz_cmd^2);
if nL <1e-4
    miu_cmd = miu_last;
else
    % atan2(y, z)，对应：
    % ny_cmd = n_lift_cmd * sin(miu_cmd)
    % nz_cmd = n_lift_cmd * cos(miu_cmd)
    miu_raw = atan2(ny_cmd, nz_cmd);
    
    % ===== 倾侧角连续化处理，避免 +pi/-pi 跳变 =====
    d_miu = miu_raw - miu_last;
    d_miu = mod(d_miu + pi, 2*pi) - pi;

    miu_cmd = miu_last + d_miu;
end
miu_cmd = mod(miu_cmd + pi, 2*pi) - pi;
% miu_cmd = -miu_cmd;
% miu_cmd = -miu_cmd;

%% ===== 攻角 =====
% C_L_alpha = (-8.19e-2)+(4.7e-2)*Ma+(1.86e-2)*alpha_deg-(4.73e-4)*(alpha_deg*Ma)-(9.19e-3)*Ma^2-(1.52e-4)*alpha_deg^2+(5.99e-7)*(alpha_deg*Ma)^2+(7.74e-4)*Ma^3+(4.08e-6)*alpha_deg^3-(2.93e-5)*Ma^4+(4.12e-7)*Ma^5;
% C_L_delta_a = (-1.45e-5)+(1.01e-4)*alpha_deg+(7.10e-6)*Ma-(4.14e-4)*delta_a-(3.51e-6)*(alpha_deg*delta_a)+(4.70e-6)*(alpha_deg*Ma)+(8.72e-6)*(Ma*delta_a)-(1.70e-7)*(alpha_deg*Ma)*delta_a;
% C_L_delta_e = (-1.45e-5)+(1.01e-4)*alpha_deg+(7.10e-6)*Ma-(4.14e-4)*delta_e-(3.51e-6)*(alpha_deg*delta_e)+(4.70e-6)*(alpha_deg*Ma)+(8.72e-6)*(Ma*delta_e)-(1.70e-7)*(alpha_deg*Ma)*delta_e;

%单位是角度
alpha_min = -30;
alpha_max = 30;

% CL_func = @(alpha_deg) (-8.19e-2)+(4.7e-2)*Ma+(1.86e-2)*alpha_deg-(4.73e-4)*(alpha_deg*Ma)-(9.19e-3)*Ma^2-(1.52e-4)*alpha_deg^2+(5.99e-7)*(alpha_deg*Ma)^2+(7.74e-4)*Ma^3+(4.08e-6)*alpha_deg^3-(2.93e-5)*Ma^4+(4.12e-7)*Ma^5 + ...
%                         (-1.45e-5)+(1.01e-4)*alpha_deg+(7.10e-6)*Ma-(4.14e-4)*delta_a-(3.51e-6)*(alpha_deg*delta_a)+(4.70e-6)*(alpha_deg*Ma)+(8.72e-6)*(Ma*delta_a)-(1.70e-7)*(alpha_deg*Ma)*delta_a + ...
%                         (-1.45e-5)+(1.01e-4)*alpha_deg+(7.10e-6)*Ma-(4.14e-4)*delta_e-(3.51e-6)*(alpha_deg*delta_e)+(4.70e-6)*(alpha_deg*Ma)+(8.72e-6)*(Ma*delta_e)-(1.70e-7)*(alpha_deg*Ma)*delta_e;

CL_func = @(alpha_deg) (-8.19e-2)+(4.7e-2)*Ma+(1.86e-2)*alpha_deg-(4.73e-4)*(alpha_deg*Ma)-(9.19e-3)*Ma^2-(1.52e-4)*alpha_deg^2+(5.99e-7)*(alpha_deg*Ma)^2+(7.74e-4)*Ma^3+(4.08e-6)*alpha_deg^3-(2.93e-5)*Ma^4+(4.12e-7)*Ma^5;
CL_min = CL_func(alpha_min);
CL_max = CL_func(alpha_max);

% ===== 目标CL =====

CL_cmd = nL*m*g/(Q*S);

% ===== 限制CL（关键）=====
CL_cmd = min(max(CL_cmd, CL_min), CL_max);

% ===== 求解 =====
alpha_cmd = fzero(@(a) CL_func(a) - CL_cmd, [alpha_min, alpha_max]);

%%

== matlab function Ctrl_For_HRV/PNG/MATLAB Function2 ==
  data: V input; f_psi output; theta input; psi input; lat input; H input
function f_psi = earth_rotation(V,theta,psi,lat,H)

earth_r = 6371000;
w_e = 7.292116000000000e-05;
R = earth_r + H;
f_psi = V*cos(theta)*sin(psi)*tan(lat)/R ...
      + 2*w_e*(sin(lat)-cos(lat)*cos(psi)*tan(theta)) ...
      + w_e^2*R*cos(lat)*sin(lat)*sin(psi)/(V*cos(theta));
